simulink model "FOC_WithHysteresis_I_Controller"  (R2018a)
settings: Solver=VariableStepAuto  StartTime=0.0  StopTime=2  MaxStep=1e-4  RelTol=1e-3
libraries: powerlib x5, simulink x1
settings Model: Creator=hp  LastModifiedBy=hp
settings DataIOCC: ReturnWorkspaceOutputs=on
settings DebuggingCC: UnconnectedInputMsg=none  UnconnectedOutputMsg=none  UnconnectedLineMsg=none
settings ModelReferenceCC: EnableRefExpFcnMdlSchedulingChecks=off
settings SFSimCC: SimUseLocalCustomCode=on
settings RTWCC: Description=Generic Real-Time Target  RTWUseLocalCustomCode=on

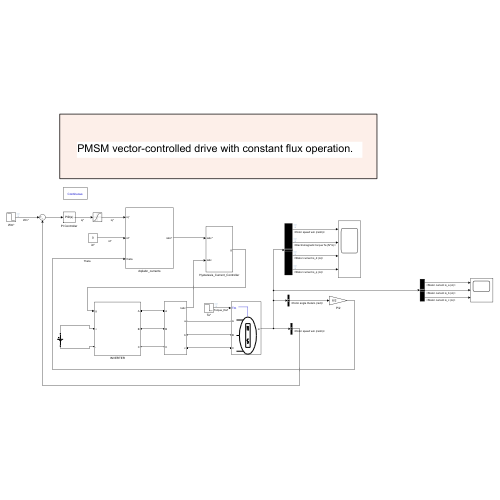
[thumbnail: Simulink's stored preview of the top-level diagram]
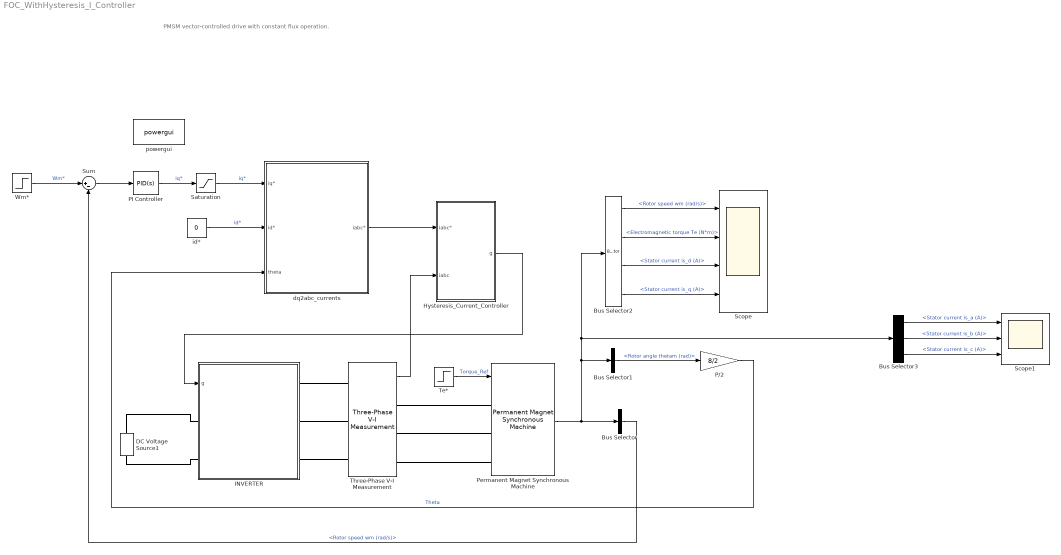
== system FOC_WithHysteresis_I_Controller ==
  note: PMSM vector-controlled drive with constant flux operation.
  Bus Selector : BusSelector  OutputSignals=Rotor speed wm (rad/s)
  Bus Selector1 : BusSelector  OutputSignals=Rotor angle thetam (rad)
  Bus Selector2 : BusSelector  OutputSignals=Rotor speed wm (rad/s),Electromagnetic torque Te (N*m),Stator current is_d (A),Stator current is_q (A)
  Bus Selector3 : BusSelector  OutputSignals=Stator current is_a (A),Stator current is_b (A),Stator current is_c (A)
  DC Voltage Source1 : powerlib/Electrical Sources/DC Voltage Source  Amplitude=400  Measurements=None
  Hysteresis_Current_Controller : Subsystem
  INVERTER : Subsystem
  P/2 : Gain  Gain=8/2
  PI Controller : simulink/Continuous/PID Controller  Controller=PID  Form=Parallel  TimeDomain=Continuous-time  SampleTime=-1  IntegratorMethod=Forward Euler  ControllerParametersSource=internal  P=1000  I=5  D=0  N=100  UseFilter=on  TunerSelectOption=Transfer Function Based (PID Tuner App)  InitialConditionSource=internal  InitialConditionForIntegrator=0  InitialConditionForFilter=0  DifferentiatorICPrevScaledInput=0  ExternalReset=none  TrackingMode=off  Kt=1  LimitOutput=off  UpperSaturationLimit=inf  LowerSaturationLimit=-inf  LinearizeAsGain=on  AntiWindupMode=none  Kb=1  POutMin=[]  POutMax=[]  IOutMin=[]  IOutMax=[]  DOutMin=[]  DOutMax=[]  NOutMin=[]  NOutMax=[]  SumOutMin=[]  SumOutMax=[]  SaturationOutMin=[]  SaturationOutMax=[]  PParamMin=[]  PParamMax=[]  IParamMin=[]  IParamMax=[]  DParamMin=[]  DParamMax=[]  NParamMin=[]  NParamMax=[]  KbParamMin=[]  KbParamMax=[]  KtParamMin=[]  KtParamMax=[]  KbOutMin=[]  KbOutMax=[]  KtOutMin=[]  KtOutMax=[]  IntegratorOutMin=[]  IntegratorOutMax=[]  FilterOutMin=[]  FilterOutMax=[]  SumI1OutMin=[]  SumI1OutMax=[]  SumI2OutMin=[]  SumI2OutMax=[]  SumI3OutMin=[]  SumI3OutMax=[]  SumDOutMin=[]  SumDOutMax=[]  DifferentiatorOutMin=[]  DifferentiatorOutMax=[]  FilterDiffOutCoefMin=[]  FilterDiffOutCoefMax=[]  ReciprocalOutMin=[]  ReciprocalOutMax=[]  SumDenOutMin=[]  SumDenOutMax=[]  SumNumOutMin=[]  SumNumOutMax=[]  DivideOutMin=[]  DivideOutMax=[]  IntegratorContinuousStateAttributes=''  IntegratorStateMustResolveToSignalObject=off  IntegratorRTWStateStorageClass=Auto  FilterContinuousStateAttributes=''  FilterStateMustResolveToSignalObject=off  FilterRTWStateStorageClass=Auto
  Permanent Magnet Synchronous Machine : powerlib/Machines/Permanent Magnet Synchronous Machine  NbPhases=3  FluxDistribution=Sinusoidal  RotorType=Salient-pole  MechanicalLoad=Torque Tm  PresetModel=No  ShowDetailedParameters=on  MeasurementBus=off  Resistance=0.4  Inductance=8.5e-3  dqInductances=[8.5e-3,8.5e-3]  La=0.000395  MachineConstant=Flux linkage established by magnets (V.s)  Flux=0.175  VoltageCst=126.966  TorqueCst=1.05  Flat=120  Mechanical=[0.0027 0.0004924 4 0]  PolePairs=4  InitialConditions=[0,0, 0,0]  InitialConditions5ph=[0 0 0 0 0 0]  RefAngle=90 degrees behind phase A axis (modified Park)  IterativeDiscreteModel=Trapezoidal non iterative  TsBlock=-1  TsPowergui=0
  Saturation : Saturate  UpperLimit=15  LowerLimit=-15
  Scope : Scope  NumInputPorts=4
  Scope1 : Scope  NumInputPorts=3
  Sum : Sum  Inputs=|+-
  Te* : Step  Before=10  After=-10  SampleTime=0
  Three-Phase V-I Measurement : powerlib/Measurements/Three-Phase V-I Measurement  VoltageMeasurement=no  SetLabelV=off  LabelV=Vabc  Vpu=off  VpuLL=off  CurrentMeasurement=yes  SetLabelI=off  LabelI=Iabc  Ipu=off  Pbase=100e6  Vbase=500e3  OutputType=Complex  PhasorSimulation=off  PSBequivalent=0
  Wm* : Step  Before=300  After=-300  SampleTime=0
  dq2abc_currents : Subsystem
  id* : Constant  Value=0
  powergui : powerlib/powergui  Priority=1  SimulationMode=Continuous  SampleTime=50e-6  frequency=60  Iterations=50  frequencyindice=0  Pbase=100e6  ErrMax=1e-4  UnitsV=kV  UnitsW=MW  buscounter=0  FunctionMessages=off  echomessages=off  EnableUseOfTLC=off  CurrentSourceSwitches=off  DisableSnubberDevices=off  DisableRonSwitches=off  DisableVfSwitches=off  DisplayEquations=off  AutomaticDiscreteSolvers=off  SolverType=Tustin/Backward Euler (TBE)  Interpol=off  ExternalGateDelay=off  methode=off  Ts=100  x0status=blocks  SPID=on  SwTol=0  HookPort=off  NonlinearTolerance=1e-4  nMaxIteration=100  ContinueOnMaxIteration=off  RestoreLinks=warning  ResistiveCurrentMeasurement=off  Frange=[0:2:500]  Ylog=off  Xlog=on  ShowGrid=off  save=off  variable=ZData  structure=0  ZoomFFT=off  StartTime=0.0  cycles=1  DisplayStyle=1  fundamental=60  FreqAxis=off  MaxFrequency=1000  frequencyindicesteady=1  RmsSteady=1  display=off
  wires:
  Sum/1 -> PI Controller/1
  Wm*/1 -> Sum/1  "Wm*"
  PI Controller/1 -> Saturation/1  "iq*"
  id*/1 -> dq2abc_currents/2(id*)  "id*"
  dq2abc_currents/1(iabc*) -> Hysteresis_Current_Controller/1(iabc*)
  Three-Phase V-I Measurement/1 -> Hysteresis_Current_Controller/2(iabc)
  Hysteresis_Current_Controller/1(g) -> INVERTER/1(g)
  Permanent Magnet Synchronous Machine/1 -> Bus Selector2/1, Bus Selector3/1, Bus Selector1/1, Bus Selector/1
  Bus Selector/1 -> Sum/2  "<Rotor speed wm (rad/s)>"
  Bus Selector1/1 -> P/2/1  "<Rotor angle thetam (rad)>"
  P/2/1 -> dq2abc_currents/3(theta)  "Theta"
  Bus Selector2/1 -> Scope/1  "<Rotor speed wm (rad/s)>"
  Bus Selector2/2 -> Scope/2  "<Electromagnetic torque Te (N*m)>"
  Bus Selector2/3 -> Scope/3  "<Stator current is_d (A)>"
  Bus Selector2/4 -> Scope/4  "<Stator current is_q (A)>"
  Te*/1 -> Permanent Magnet Synchronous Machine/1  "Torque_Ref"
  Saturation/1 -> dq2abc_currents/1(iq*)  "iq*"
  Bus Selector3/2 -> Scope1/2  "<Stator current is_b (A)>"
  Bus Selector3/1 -> Scope1/1  "<Stator current is_a (A)>"
  Bus Selector3/3 -> Scope1/3  "<Stator current is_c (A)>"
  connections:
  Three-Phase V-I Measurement/LConn1 -- INVERTER/RConn1
  INVERTER/RConn2 -- Three-Phase V-I Measurement/LConn2
  INVERTER/RConn3 -- Three-Phase V-I Measurement/LConn3
  Permanent Magnet Synchronous Machine/LConn3 -- Three-Phase V-I Measurement/RConn3
  Permanent Magnet Synchronous Machine/LConn1 -- Three-Phase V-I Measurement/RConn1
  Permanent Magnet Synchronous Machine/LConn2 -- Three-Phase V-I Measurement/RConn2
  DC Voltage Source1/RConn1 -- INVERTER/LConn1
  INVERTER/LConn2 -- DC Voltage Source1/LConn1

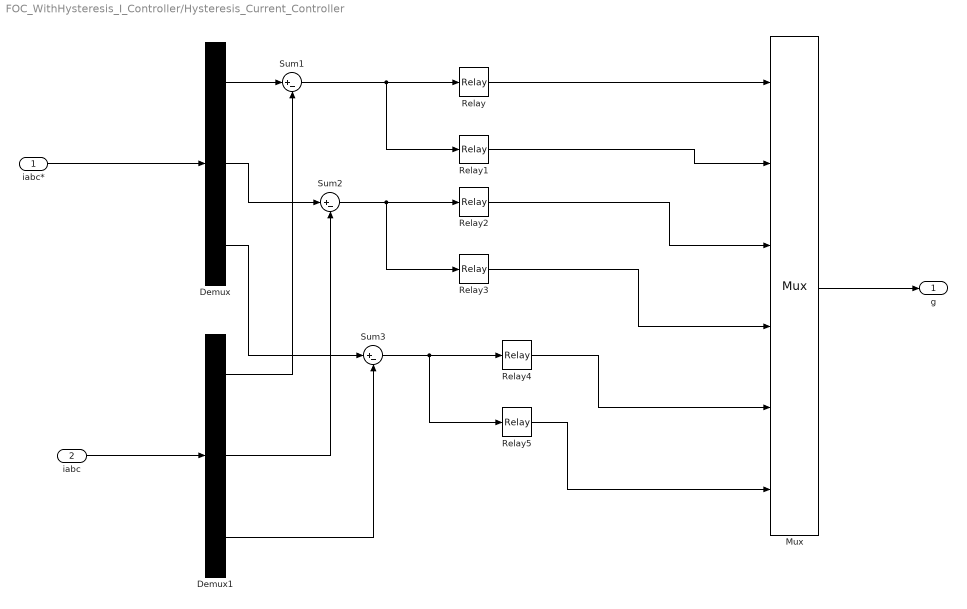
== system FOC_WithHysteresis_I_Controller/Hysteresis_Current_Controller ==
  iabc* : Inport
  iabc : Inport  Port=2
  Demux : Demux  Outputs=3
  Demux1 : Demux  Outputs=3
  Mux : Mux  Inputs=6
  Relay : Relay  OnSwitchValue=0.01  OffSwitchValue=-0.01
  Relay1 : Relay  OnSwitchValue=0.01  OffSwitchValue=-0.01  OnOutputValue=0  OffOutputValue=1
  Relay2 : Relay  OnSwitchValue=0.01  OffSwitchValue=-0.01
  Relay3 : Relay  OnSwitchValue=0.01  OffSwitchValue=-0.01  OnOutputValue=0  OffOutputValue=1
  Relay4 : Relay  OnSwitchValue=0.01  OffSwitchValue=-0.01
  Relay5 : Relay  OnSwitchValue=0.01  OffSwitchValue=-0.01  OnOutputValue=0  OffOutputValue=1
  Sum1 : Sum  Inputs=|+-
  Sum2 : Sum  Inputs=|+-
  Sum3 : Sum  Inputs=|+-
  g : Outport
  wires:
  Sum2/1 -> Relay2/1, Relay3/1
  Relay3/1 -> Mux/4
  Demux1/2 -> Sum2/2
  Sum3/1 -> Relay5/1, Relay4/1
  Relay4/1 -> Mux/5
  Sum1/1 -> Relay1/1, Relay/1
  Demux/1 -> Sum1/1
  Relay/1 -> Mux/1
  Relay5/1 -> Mux/6
  iabc/1 -> Demux1/1
  Mux/1 -> g/1
  Demux/2 -> Sum2/1
  iabc*/1 -> Demux/1
  Demux/3 -> Sum3/1
  Demux1/1 -> Sum1/2
  Relay1/1 -> Mux/2
  Demux1/3 -> Sum3/2
  Relay2/1 -> Mux/3

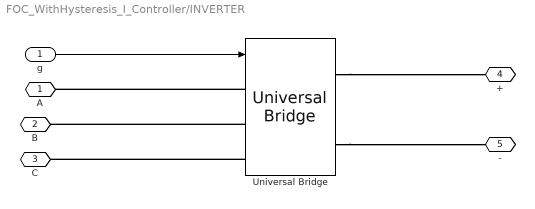
== system FOC_WithHysteresis_I_Controller/INVERTER ==
  g : Inport
  Universal Bridge : powerlib/Power Electronics/Universal Bridge  Arms=3  SnubberResistance=1e5  SnubberCapacitance=inf  Device=IGBT / Diodes  Ron=1e-3  Lon=0  ForwardVoltages="[  0  0  ]"  ForwardVoltage=0  GTOparameters=[ 10e-6 , 20e-6 ]  IGBTparameters=[ 1e-6 , 2e-6 ]  Measurements=None  Measurements_2=None  converterType=Rectifier
  A : PMIOPort  Side=Right
  B : PMIOPort  Port=2  Side=Right
  C : PMIOPort  Port=3  Side=Right
  + : PMIOPort  Port=4  Side=Left
  - : PMIOPort  Port=5  Side=Left
  wires:
  g/1 -> Universal Bridge/1
  connections:
  Universal Bridge/RConn1 -- +/RConn1
  Universal Bridge/LConn3 -- C/RConn1
  Universal Bridge/LConn2 -- B/RConn1
  Universal Bridge/LConn1 -- A/RConn1
  Universal Bridge/RConn2 -- -/RConn1

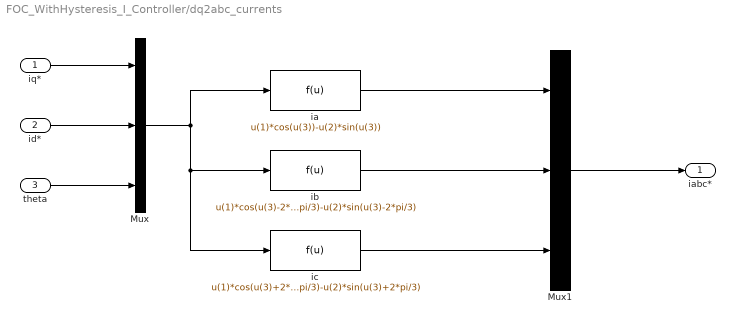
== system FOC_WithHysteresis_I_Controller/dq2abc_currents ==
  iq* : Inport
  id* : Inport  Port=2
  theta : Inport  Port=3
  Mux : Mux  Inputs=3
  Mux1 : Mux  Inputs=3
  ia : Fcn  Expr=u(1)*cos(u(3))-u(2)*sin(u(3))
  ib : Fcn  Expr=u(1)*cos(u(3)-2*pi/3)-u(2)*sin(u(3)-2*pi/3)
  ic : Fcn  Expr=u(1)*cos(u(3)+2*pi/3)-u(2)*sin(u(3)+2*pi/3)
  iabc* : Outport
  wires:
  Mux/1 -> ia/1, ic/1, ib/1
  ic/1 -> Mux1/3
  iq*/1 -> Mux/1
  ia/1 -> Mux1/1
  id*/1 -> Mux/2
  ib/1 -> Mux1/2
  theta/1 -> Mux/3
  Mux1/1 -> iabc*/1
